simulink model "DFIG_Dynamic_Model"  (R2013a)
settings: Solver=ode45  StartTime=0.0  StopTime=25  RelTol=1e-3
values from neighbouring files (symbols this model uses):
  B = inv([ ... (first row only)    [WECSConstants.m]
  C = 14e-3    (= 0.014)    [WECSConstants.m]
  f = 60    [WECSConstants.m]
  Ib = Pb/Vb    (= 1673.47904113)    [WECSConstants.m]
  Kf = 5    [WECSConstants.m]
  Ki = 1    [WECSConstants.m]
  Kp = 3    [WECSConstants.m]
  Lg = Xg/wb    (= 0.000189434171015)    [WECSConstants.m]
  Lm = Xm/wb    (= 0.00249597832282)    [WECSConstants.m]
  Lr = Xr/wb    (= 0.00255883889524)    [WECSConstants.m]
  Ls = Xs/wb    (= 0.00255426721724)    [WECSConstants.m]
  P = 6    [WECSConstants.m]
  Pb = (2e6)/3    (= 666666.666667)    [WECSConstants.m]
  sigma = 1-(Lm*Lm)/(Ls*Lr)    (= 0.0468256531123)    [WECSConstants.m]
  Tcomp = 1    [WECSConstants.m]
  Ts = 5e-5    (= 5e-05)    [WECSConstants.m]
  Vb = 690/(3^0.5)    (= 398.371685741)    [WECSConstants.m]
  VDC0 = 1200    [WECSConstants.m]
  wb = 2*pi*f    (= 376.991118431)    [WECSConstants.m]
  ws = wb    (= 376.991118431)    [WECSConstants.m]
  Xm_pu = 3.95279    [WECSConstants.m]
  Xr_pu = Xlr_pu+Xm_pu    (= 4.05234)    [WECSConstants.m]
  Z = [ ... (first row only)    [WECSConstants.m]
  Zb = Vb/Ib    (= 0.23805)    [WECSConstants.m]
undefined symbols (not defined in the file or in its folder): i
libraries: powerlib_extras x13, powerlib_meascontrol x2
(part 2 of 2)

== system DFIG_Dynamic_Model/RSC Control/Negative RSC Control/dq+ // dq-2/LPF1 ==
  I : Inport
  Gain : Gain  Gain=Kf
  Gain1 : Gain  Gain=Kf
  Integrator : Integrator
  Sum : Sum  Inputs=|+-
  O : Outport
  wires:
  Sum/1 -> Integrator/1
  Integrator/1 -> O/1, Gain/1
  I/1 -> Gain1/1
  Gain/1 -> Sum/2
  Gain1/1 -> Sum/1

== system DFIG_Dynamic_Model/RSC Control/Negative RSC Control/dq+ // dq-2/LPF3 ==
  I : Inport
  Gain : Gain  Gain=Kf
  Gain1 : Gain  Gain=Kf
  Integrator : Integrator
  Sum : Sum  Inputs=|+-
  O : Outport
  wires:
  Sum/1 -> Integrator/1
  Integrator/1 -> O/1, Gain/1
  I/1 -> Gain1/1
  Gain/1 -> Sum/2
  Gain1/1 -> Sum/1

== system DFIG_Dynamic_Model/RSC Control/Negative RSC Control/dq+ // dq-3/LPF1 ==
  I : Inport
  Gain : Gain  Gain=Kf
  Gain1 : Gain  Gain=Kf
  Integrator : Integrator
  Sum : Sum  Inputs=|+-
  O : Outport
  wires:
  Sum/1 -> Integrator/1
  Integrator/1 -> O/1, Gain/1
  I/1 -> Gain1/1
  Gain/1 -> Sum/2
  Gain1/1 -> Sum/1

== system DFIG_Dynamic_Model/RSC Control/Negative RSC Control/dq+ // dq-3/LPF2 ==
  I : Inport
  Gain : Gain  Gain=Kf
  Gain1 : Gain  Gain=Kf
  Integrator : Integrator
  Sum : Sum  Inputs=|+-
  O : Outport
  wires:
  Sum/1 -> Integrator/1
  Integrator/1 -> O/1, Gain/1
  I/1 -> Gain1/1
  Gain/1 -> Sum/2
  Gain1/1 -> Sum/1

== system DFIG_Dynamic_Model/RSC Control/Negative RSC Control/dq+ // dq-3/LPF3 ==
  I : Inport
  Gain : Gain  Gain=Kf
  Gain1 : Gain  Gain=Kf
  Integrator : Integrator
  Sum : Sum  Inputs=|+-
  O : Outport
  wires:
  Sum/1 -> Integrator/1
  Integrator/1 -> O/1, Gain/1
  I/1 -> Gain1/1
  Gain/1 -> Sum/2
  Gain1/1 -> Sum/1

== system DFIG_Dynamic_Model/RSC Control/Negative RSC Control/dq- // dq+/LPF1 ==
  I : Inport
  Gain : Gain  Gain=Kf
  Gain1 : Gain  Gain=Kf
  Integrator : Integrator
  Sum : Sum  Inputs=|+-
  O : Outport
  wires:
  Sum/1 -> Integrator/1
  Integrator/1 -> O/1, Gain/1
  I/1 -> Gain1/1
  Gain/1 -> Sum/2
  Gain1/1 -> Sum/1

== system DFIG_Dynamic_Model/RSC Control/Negative RSC Control/dq- // dq+/LPF3 ==
  I : Inport
  Gain : Gain  Gain=Kf
  Gain1 : Gain  Gain=Kf
  Integrator : Integrator
  Sum : Sum  Inputs=|+-
  O : Outport
  wires:
  Sum/1 -> Integrator/1
  Integrator/1 -> O/1, Gain/1
  I/1 -> Gain1/1
  Gain/1 -> Sum/2
  Gain1/1 -> Sum/1
